simulink model "controller"  (R2018b)
settings: Solver=FixedStepAuto  StartTime=0.0  StopTime=20  FixedStep=1/100  RelTol=1e-3
settings Model: Creator=pthb3  LastModifiedBy=pthb3

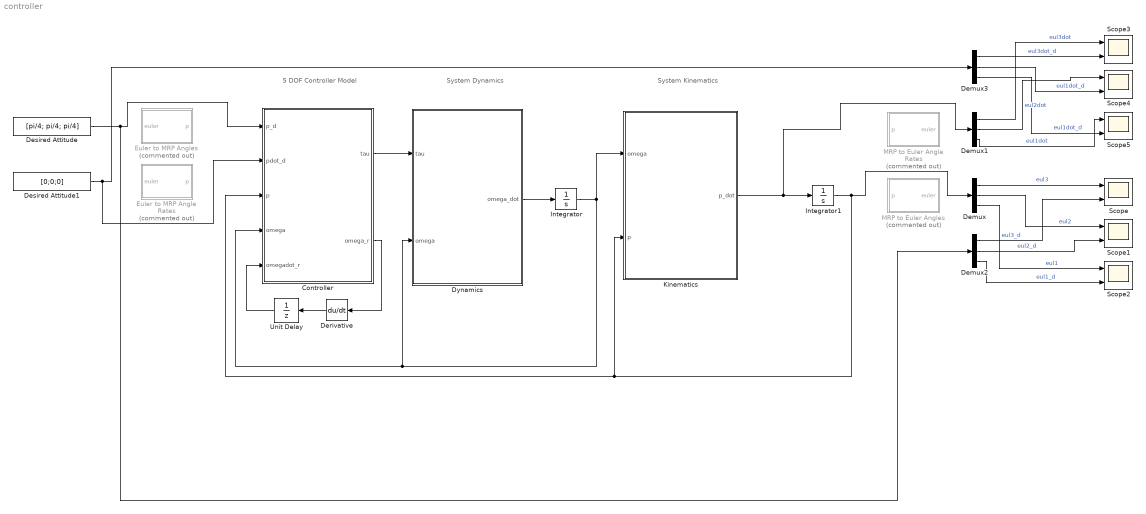
== system controller ==
  note: System
      | Kinematics
  note: System
      | Dynamics
  note: 5 DOF
      | Controller Model
  Controller : MATLAB Function  TreatAsAtomicUnit=on
  Demux{,1..3} (4 alike) : Demux  Outputs=3
  Derivative : Derivative
  Desired Attitude : Constant  Value=[pi/4; pi/4; pi/4]
  Desired Attitude1 : Constant  Value=[0;0;0]
  Dynamics : MATLAB Function  TreatAsAtomicUnit=on
  Euler to MRP Angle Rates : MATLAB Function  Commented=on  TreatAsAtomicUnit=on
  Euler to MRP Angles : MATLAB Function  Commented=on  TreatAsAtomicUnit=on
  Integrator : Integrator  InitialCondition=[0;0;0]
  Integrator1 : Integrator  InitialCondition=[0;0;0];
  Kinematics : MATLAB Function  TreatAsAtomicUnit=on
  MRP to Euler Angle Rates : MATLAB Function  Commented=on  TreatAsAtomicUnit=on
  MRP to Euler Angles : MATLAB Function  Commented=on  TreatAsAtomicUnit=on
  Scope{,1..5} (6 alike) : Scope  NumInputPorts=2
  Unit Delay : UnitDelay  InitialCondition=[0;0;0]  SampleTime=-1
  wires:
  Kinematics/1(p_dot) -> Demux1/1, Integrator1/1
  Dynamics/1(omega_dot) -> Integrator/1
  Integrator/1 -> Dynamics/2(omega), Controller/4(omega), Kinematics/1(omega)
  Integrator1/1 -> Demux/1, Controller/3(p), Kinematics/2(p)
  Controller/2(omega_r) -> Derivative/1
  Derivative/1 -> Unit Delay/1
  Controller/1(tau) -> Dynamics/1(tau)
  Demux/1 -> Scope/1  "eul3"
  Demux/2 -> Scope1/1  "eul2"
  Demux/3 -> Scope2/1  "eul1"
  Desired Attitude1/1 -> Controller/2(pdot_d), Demux3/1
  Demux2/1 -> Scope/2  "eul3_d"
  Demux2/2 -> Scope1/2  "eul2_d"
  Demux2/3 -> Scope2/2  "eul1_d"
  Demux1/1 -> Scope3/1  "eul3dot"
  Demux1/2 -> Scope4/1  "eul2dot"
  Demux1/3 -> Scope5/1  "eul1dot"
  Demux3/1 -> Scope3/2  "eul3dot_d"
  Demux3/2 -> Scope4/2  "eul1dot_d"
  Demux3/3 -> Scope5/2  "eul1dot_d"
  Desired Attitude/1 -> Demux2/1, Controller/1(p_d)
  Unit Delay/1 -> Controller/5(omegadot_r)

== matlab function controller/Dynamics ==
  data: omega_dot output; tau input; omega input
function omega_dot = dynamics(tau, omega)

S = @(p) [0, -p(3), p(2); p(3) 0 -p(1); -p(2) p(1) 0];

% Model Parameters
J = eye(3); % Inertia matrix
M_b = J; % Eqn (6), should just be J
C_b = -S(J*omega); % Eqn (6), should just be -S(J*omega)
H_b = zeros(3,1); % Eqn 8

omega_dot = inv(M_b) * (tau - C_b*omega - H_b); % Eqn (5)

== matlab function controller/Controller ==
  data: tau output; p_d input; pdot_d input; p input; omega input; omegadot_r input; omega_r output
function [tau, omega_r] = controller(p_d, pdot_d, p, omega, omegadot_r)

% Controller Gains
Lambda = eye(3); % Controller Gain
K_omega = eye(3); % Controller Gain

% Eqn (2)
I_3 = eye(3);
S = @(p) [0, -p(3), p(2); p(3) 0 -p(1); -p(2) p(1) 0];
Z = @(p) 1/2 * ( I_3*(1-p'*p)/2 + p*p' + S(p) );

% Model Parameters
J = eye(3); % Inertia matrix
M_b = J; % Eqn (6), should just be J
C_b = -S(J*omega); % Eqn (6), should just be -S(J*omega)
H_b = zeros(3,1); % Eqn 8

% Eqn (9) funnction of p, p_d, pdot_d
omega_r = (inv(Z(p)) * pdot_d) + (inv(Z(p)) * Lambda * (p_d - p));

% above Eqn (9)
s_omega = omega - omega_r;

% Eqn (10) function of omega_r, omega_r_dot, s_omega, K_omega
tau = M_b*omegadot_r + C_b*omega_r + H_b - K_omega*s_omega;

== matlab function controller/Kinematics ==
  data: omega input; p_dot output; p input
function p_dot = kinematics(omega, p)

% Eqn (2)
I_3 = eye(3);
S = @(p) [0, -p(3), p(2); p(3) 0 -p(1); -p(2) p(1) 0];
Z = @(p) 1/2 * ( I_3*(1-p'*p)/2 + p*p' + S(p) );

p_dot = Z(p) * omega; % Eqn (2)

== matlab function controller/MRP to Euler Angles ==
  data: p input; euler output
function euler = mrp2euler(p)

euler = ConvertAttitude(p, 'mrp', '321');

== matlab function controller/Euler to MRP Angles ==
  data: euler input; p output
function p = euler2mrp(euler)

p = ConvertAttitude(euler, '321', 'mrp');

== matlab function controller/MRP to Euler Angle Rates ==
  data: p input; euler output
function euler = mrp2euler(p)

euler = ConvertAttitude(p, 'mrp', '321');

== matlab function controller/Euler to MRP Angle Rates ==
  data: euler input; p output
function p = euler2mrp(euler)

p = ConvertAttitude(euler, '321', 'mrp');
